simulink model "lti_simulink"  (R2015a)
settings: Solver=ode45  StartTime=0.0  StopTime=10.0  RelTol=1e-3
settings Model: Creator=patel  LastModifiedBy=patel

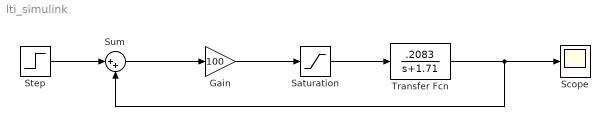
== system lti_simulink ==
  Gain : Gain  Gain=100
  Saturation : Saturate  UpperLimit=5  LowerLimit=5
  Scope : Scope
  Step : Step  After=10  SampleTime=0
  Sum : Sum  Inputs=|++
  Transfer Fcn : TransferFcn  Numerator=[.2083]  Denominator=[1 1.71]
  wires:
  Step/1 -> Sum/1
  Sum/1 -> Gain/1
  Gain/1 -> Saturation/1
  Saturation/1 -> Transfer Fcn/1
  Transfer Fcn/1 -> Sum/2, Scope/1
